simulink model "VCO_15N_2nd_order_2020a_v2"  (R2020b)
settings: Solver=VariableStepAuto  StartTime=0.0  StopTime=5000*clk_p  RelTol=1e-3
values from neighbouring files (symbols this model uses):
  clk_p = 1/clk    (= 5e-09)    [parallel_simulink_test8.m]
  finw = 2*pi*M/(N_in*clk_p)    (= 3374757.73335)    [parallel_simulink_test8.m]
undefined symbols (not defined in the file or in its folder): Amp_in, Bias, gain_DAC
libraries: commsynccomp2 x60, simulink_extras x9, eeGeneralControl x3
(part 1 of 2)
settings Model: SimulationMode=accelerator  Creator=97826  LastModifiedBy=97826
settings SFSimCC: CustomCodeUndefinedFunction=UseInterfaceOnly

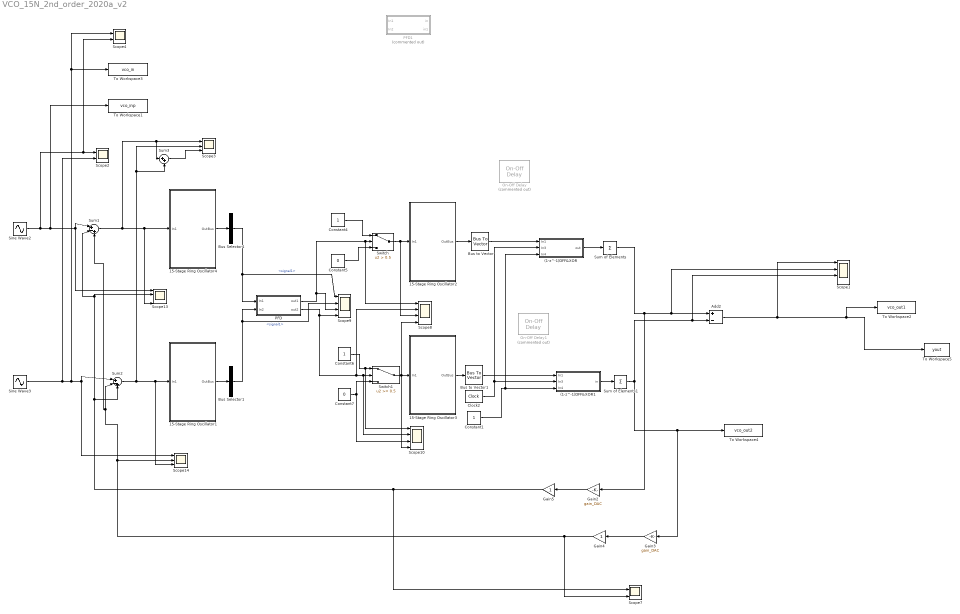
== system VCO_15N_2nd_order_2020a_v2 ==
  (1-z^-1)DFF&XOR : Subsystem  TreatAsAtomicUnit=on
  (1-z^-1)DFF&XOR1 : Subsystem  TreatAsAtomicUnit=on
  15-Stage Ring Oscillator1 : Subsystem
  15-Stage Ring Oscillator2 : Subsystem
  15-Stage Ring Oscillator3 : Subsystem
  15-Stage Ring Oscillator4 : Subsystem
  Add2 : Sum  Inputs=+-
  Bus Selector1 : BusSelector  OutputSignals=signal1
  Bus Selector4 : BusSelector  OutputSignals=signal1
  Bus to Vector : BusToVector
  Bus to Vector1 : BusToVector
  Clock2 : simulink_extras/Flip Flops/Clock  period=clk_p
  Constant1 : Constant
  Constant4 : Constant
  Constant5 : Constant  Value=0
  Constant6 : Constant
  Constant7 : Constant  Value=0
  Gain2 : Gain  Gain=gain_DAC
  Gain3 : Gain  Gain=gain_DAC
  Gain4 : Gain
  Gain5 : Gain
  On-Off Delay : eeGeneralControl/On-Off Delay  Commented=on  LabelModeActiveChoice=Continuous  Td_on=1500e-12  Td_off=1500e-12  IC=0  Ts=0
      settings: SourceProductBaseCode=PS
  On-Off Delay1 : eeGeneralControl/On-Off Delay  Commented=on  LabelModeActiveChoice=Continuous  Td_on=1500e-12  Td_off=1500e-12  IC=0  Ts=0
      settings: SourceProductBaseCode=PS
  PFD : Subsystem  TreatAsAtomicUnit=on
  PFD1 : Subsystem  Commented=on  TreatAsAtomicUnit=on
  Scope{1,8..10,13} (5 alike) : Scope  NumInputPorts=4
  Scope14 : Scope  NumInputPorts=3
  Scope2 : Scope  NumInputPorts=2
  Scope3 : Scope  NumInputPorts=3
  Scope4 : Scope  NumInputPorts=2
  Scope7 : Scope  NumInputPorts=2
  Sine Wave2 : Sin  Amplitude=Amp_in  Bias=Bias  Frequency=finw  SampleTime=0
  Sine Wave3 : Sin  Amplitude=Amp_in  Bias=Bias  Frequency=finw  Phase=pi  SampleTime=0
  Sum of Elements : Sum  Inputs=+  CollapseMode=Specified dimension
  Sum of Elements1 : Sum  Inputs=+  CollapseMode=Specified dimension
  Sum1 : Sum  Inputs=|+-+
  Sum2 : Sum  Inputs=|+-+
  Sum3 : Sum  Inputs=|++
  Switch : Switch  Criteria=u2 > Threshold  Threshold=0.5
  Switch1 : Switch  Threshold=0.5
  To Workspace1 : ToWorkspace  VariableName=vco_inp  SampleTime=-1
  To Workspace2 : ToWorkspace  VariableName=vco_out1  SampleTime=clk_p
  To Workspace3 : ToWorkspace  VariableName=vco_in  SampleTime=-1
  To Workspace4 : ToWorkspace  VariableName=vco_out2  SampleTime=-1
  To Workspace5 : ToWorkspace  VariableName=yout  SampleTime=-1
  wires:
  Sum2/1 -> 15-Stage Ring Oscillator1/1(In1), Scope14/3, Sum3/2, Scope3/2
  Sine Wave3/1 -> Scope4/1, To Workspace3/1, Scope14/1, Sum2/1, Scope2/2
  Gain5/1 -> Sum2/3, Sum1/2, Scope13/2, Scope7/1
  Sine Wave2/1 -> Scope4/2, Scope2/1, To Workspace1/1, Scope13/1, Sum1/1
  Gain4/1 -> Sum1/3, Sum2/2, Scope14/2, Scope7/2
  Gain3/1 -> Gain4/1
  Gain2/1 -> Gain5/1
  Sum1/1 -> Sum3/1, Scope3/1, Scope13/4, 15-Stage Ring Oscillator4/1(In1)
  15-Stage Ring Oscillator4/1(OutBus) -> Bus Selector4/1
  Bus Selector4/1 -> PFD/1(In1), Scope9/1  "<signal1>"
  Bus Selector1/1 -> Scope9/2, PFD/2(In2)  "<signal1>"
  15-Stage Ring Oscillator1/1(OutBus) -> Bus Selector1/1
  Switch/1 -> Scope8/3, 15-Stage Ring Oscillator2/1(In1)
  Constant4/1 -> Switch/1
  Constant5/1 -> Switch/3
  PFD/1(out1) -> Scope9/3, Scope8/1, Switch/2
  Switch1/1 -> 15-Stage Ring Oscillator3/1(In1), Scope8/4, Scope10/4
  Constant7/1 -> Scope10/3, Switch1/3
  Constant6/1 -> Scope10/1, Switch1/1
  PFD/2(out2) -> Scope9/4, Scope8/2, Scope10/2, Switch1/2
  Clock2/1 -> (1-z^-1)DFF&XOR/2(In3), (1-z^-1)DFF&XOR1/2(In3)
  Constant1/1 -> (1-z^-1)DFF&XOR/3(In4), (1-z^-1)DFF&XOR1/3(In4)
  (1-z^-1)DFF&XOR/1(out) -> Sum of Elements/1
  (1-z^-1)DFF&XOR1/1(in) -> Sum of Elements1/1
  Sum of Elements/1 -> Gain2/1, Scope1/2, Add2/1
  Sum of Elements1/1 -> Gain3/1, To Workspace4/1, Scope1/3, Add2/2
  15-Stage Ring Oscillator3/1(OutBus) -> Bus to Vector1/1
  Add2/1 -> Scope1/1, To Workspace2/1, To Workspace5/1
  Sum3/1 -> Scope3/3
  15-Stage Ring Oscillator2/1(OutBus) -> Bus to Vector/1
  Bus to Vector/1 -> (1-z^-1)DFF&XOR/1(In1)
  Bus to Vector1/1 -> (1-z^-1)DFF&XOR1/1(In1)

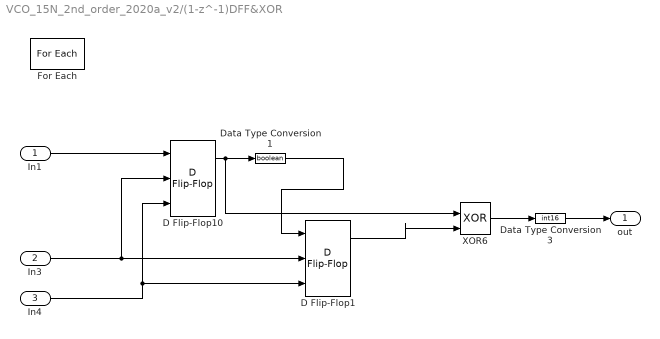
== system VCO_15N_2nd_order_2020a_v2/(1-z^-1)DFF&XOR ==
  In1 : Inport  Partition=on  PartitionDimension=1  PartitionWidth=N_stage  PartitionOffset=0
  In3 : Inport  Port=2
  In4 : Inport  Port=3
  D Flip-Flop1 : simulink_extras/Flip Flops/D Flip-Flop
  D Flip-Flop10 : simulink_extras/Flip Flops/D Flip-Flop
  Data Type Conversion1 : DataTypeConversion  OutDataTypeStr=boolean
  Data Type Conversion3 : DataTypeConversion  OutDataTypeStr=int16
  For Each : ForEach  DisableCoverage=on
  XOR6 : Logic  Operator=XOR  IconShape=distinctive  AllPortsSameDT=off  OutDataTypeStr=boolean
  out : Outport  ConcatenationDimension=1
  wires:
  In3/1 -> D Flip-Flop10/2, D Flip-Flop1/2
  In4/1 -> D Flip-Flop10/3, D Flip-Flop1/3
  Data Type Conversion3/1 -> out/1
  XOR6/1 -> Data Type Conversion3/1
  D Flip-Flop1/1 -> XOR6/2
  In1/1 -> D Flip-Flop10/1
  D Flip-Flop10/1 -> XOR6/1, Data Type Conversion1/1
  Data Type Conversion1/1 -> D Flip-Flop1/1

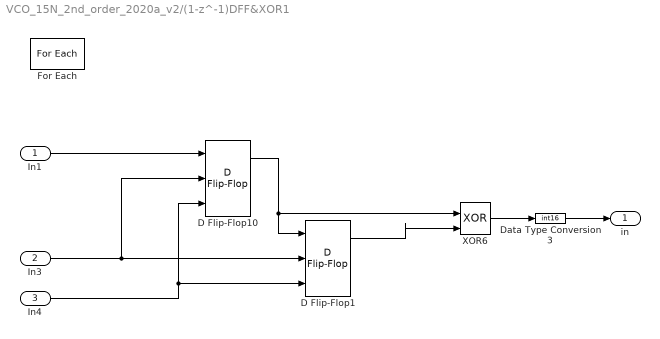
== system VCO_15N_2nd_order_2020a_v2/(1-z^-1)DFF&XOR1 ==
  In1 : Inport  Partition=on  PartitionDimension=1  PartitionWidth=N_stage  PartitionOffset=0
  In3 : Inport  Port=2
  In4 : Inport  Port=3
  D Flip-Flop1 : simulink_extras/Flip Flops/D Flip-Flop
  D Flip-Flop10 : simulink_extras/Flip Flops/D Flip-Flop
  Data Type Conversion3 : DataTypeConversion  OutDataTypeStr=int16
  For Each : ForEach  DisableCoverage=on
  XOR6 : Logic  Operator=XOR  IconShape=distinctive  AllPortsSameDT=off  OutDataTypeStr=boolean
  in : Outport  ConcatenationDimension=1
  wires:
  In3/1 -> D Flip-Flop10/2, D Flip-Flop1/2
  In4/1 -> D Flip-Flop10/3, D Flip-Flop1/3
  Data Type Conversion3/1 -> in/1
  In1/1 -> D Flip-Flop10/1
  XOR6/1 -> Data Type Conversion3/1
  D Flip-Flop1/1 -> XOR6/2
  D Flip-Flop10/1 -> XOR6/1, D Flip-Flop1/1

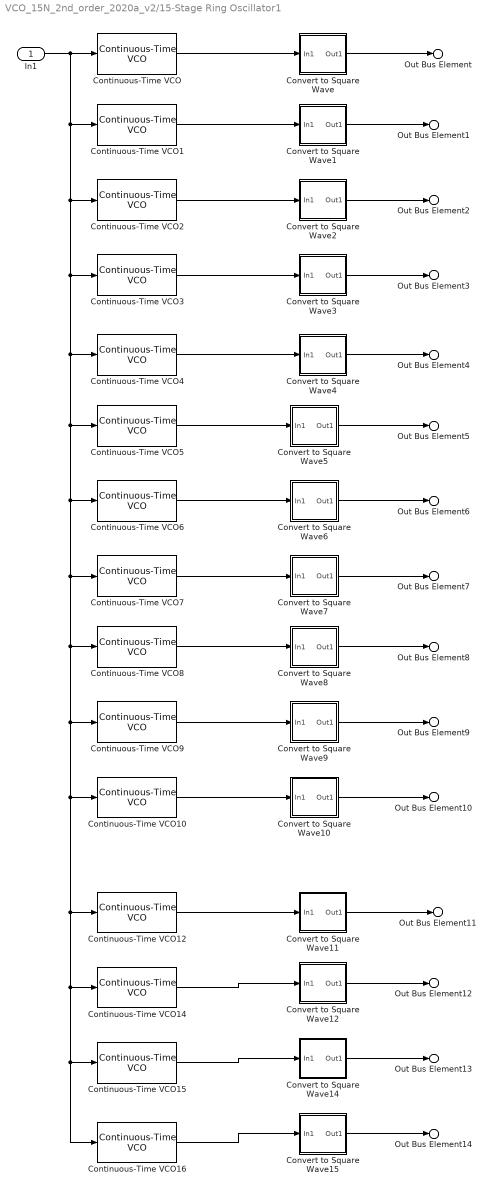
== system VCO_15N_2nd_order_2020a_v2/15-Stage Ring Oscillator1 ==
  In1 : Inport
  Continuous-Time VCO : commsynccomp2/Continuous-Time VCO  Ac=1  Fc=VCO_center_freq1  Kc=KVCO  Ph=1
      settings: SourceProductBaseCode=CM
  Continuous-Time VCO1 : commsynccomp2/Continuous-Time VCO  Ac=1  Fc=VCO_center_freq1  Kc=KVCO  Ph=pi-pi/15+1
      settings: SourceProductBaseCode=CM
  Continuous-Time VCO10 : commsynccomp2/Continuous-Time VCO  Ac=1  Fc=VCO_center_freq1  Kc=KVCO  Ph=-10*pi/15+1
      settings: SourceProductBaseCode=CM
  Continuous-Time VCO12 : commsynccomp2/Continuous-Time VCO  Ac=1  Fc=VCO_center_freq1  Kc=KVCO  Ph=pi-11*pi/15+1
      settings: SourceProductBaseCode=CM
  Continuous-Time VCO14 : commsynccomp2/Continuous-Time VCO  Ac=1  Fc=VCO_center_freq1  Kc=KVCO  Ph=-12*pi/15+1
      settings: SourceProductBaseCode=CM
  Continuous-Time VCO15 : commsynccomp2/Continuous-Time VCO  Ac=1  Fc=VCO_center_freq1  Kc=KVCO  Ph=pi-13*pi/15+1
      settings: SourceProductBaseCode=CM
  Continuous-Time VCO16 : commsynccomp2/Continuous-Time VCO  Ac=1  Fc=VCO_center_freq1  Kc=KVCO  Ph=-14*pi/15+1
      settings: SourceProductBaseCode=CM
  Continuous-Time VCO2 : commsynccomp2/Continuous-Time VCO  Ac=1  Fc=VCO_center_freq1  Kc=KVCO  Ph=-2*pi/15+1
      settings: SourceProductBaseCode=CM
  Continuous-Time VCO3 : commsynccomp2/Continuous-Time VCO  Ac=1  Fc=VCO_center_freq1  Kc=KVCO  Ph=pi-3*pi/15+1
      settings: SourceProductBaseCode=CM
  Continuous-Time VCO4 : commsynccomp2/Continuous-Time VCO  Ac=1  Fc=VCO_center_freq1  Kc=KVCO  Ph=-4*pi/15+1
      settings: SourceProductBaseCode=CM
  Continuous-Time VCO5 : commsynccomp2/Continuous-Time VCO  Ac=1  Fc=VCO_center_freq1  Kc=KVCO  Ph=pi-5*pi/15+1
      settings: SourceProductBaseCode=CM
  Continuous-Time VCO6 : commsynccomp2/Continuous-Time VCO  Ac=1  Fc=VCO_center_freq1  Kc=KVCO  Ph=-6*pi/15+1
      settings: SourceProductBaseCode=CM
  Continuous-Time VCO7 : commsynccomp2/Continuous-Time VCO  Ac=1  Fc=VCO_center_freq1  Kc=KVCO  Ph=pi-7*pi/15+1
      settings: SourceProductBaseCode=CM
  Continuous-Time VCO8 : commsynccomp2/Continuous-Time VCO  Ac=1  Fc=VCO_center_freq1  Kc=KVCO  Ph=-8*pi/15+1
      settings: SourceProductBaseCode=CM
  Continuous-Time VCO9 : commsynccomp2/Continuous-Time VCO  Ac=1  Fc=VCO_center_freq1  Kc=KVCO  Ph=pi-9*pi/15+1
      settings: SourceProductBaseCode=CM
  Convert to Square Wave : Subsystem
  Convert to Square Wave1 : Subsystem
  Convert to Square Wave10 : Subsystem
  Convert to Square Wave11 : Subsystem
  Convert to Square Wave12 : Subsystem
  Convert to Square Wave14 : Subsystem
  Convert to Square Wave15 : Subsystem
  Convert to Square Wave2 : Subsystem
  Convert to Square Wave3 : Subsystem
  Convert to Square Wave4 : Subsystem
  Convert to Square Wave5 : Subsystem
  Convert to Square Wave6 : Subsystem
  Convert to Square Wave7 : Subsystem
  Convert to Square Wave8 : Subsystem
  Convert to Square Wave9 : Subsystem
  Out Bus Element : Outport  PortName=OutBus  Element=signal1
  Out Bus Element1 : Outport  PortName=OutBus  Element=signal2
  Out Bus Element2 : Outport  PortName=OutBus  Element=signal3
  Out Bus Element3 : Outport  PortName=OutBus  Element=signal4
  Out Bus Element4 : Outport  PortName=OutBus  Element=signal5
  Out Bus Element5 : Outport  PortName=OutBus  Element=signal6
  Out Bus Element6 : Outport  PortName=OutBus  Element=signal7
  Out Bus Element7 : Outport  PortName=OutBus  Element=signal8
  Out Bus Element8 : Outport  PortName=OutBus  Element=signal9
  Out Bus Element9 : Outport  PortName=OutBus  Element=signal10
  Out Bus Element10 : Outport  PortName=OutBus  Element=signal11
  Out Bus Element11 : Outport  PortName=OutBus  Element=signal12
  Out Bus Element12 : Outport  PortName=OutBus  Element=signal13
  Out Bus Element13 : Outport  PortName=OutBus  Element=signal14
  Out Bus Element14 : Outport  PortName=OutBus  Element=signal15
  wires:
  Continuous-Time VCO/1 -> Convert to Square Wave/1(In1)
  Continuous-Time VCO1/1 -> Convert to Square Wave1/1(In1)
  Continuous-Time VCO2/1 -> Convert to Square Wave2/1(In1)
  Continuous-Time VCO3/1 -> Convert to Square Wave3/1(In1)
  Continuous-Time VCO4/1 -> Convert to Square Wave4/1(In1)
  Continuous-Time VCO5/1 -> Convert to Square Wave5/1(In1)
  Continuous-Time VCO6/1 -> Convert to Square Wave6/1(In1)
  Continuous-Time VCO7/1 -> Convert to Square Wave7/1(In1)
  Continuous-Time VCO8/1 -> Convert to Square Wave8/1(In1)
  Continuous-Time VCO9/1 -> Convert to Square Wave9/1(In1)
  Continuous-Time VCO10/1 -> Convert to Square Wave10/1(In1)
  Convert to Square Wave/1(Out1) -> Out Bus Element/1
  Convert to Square Wave1/1(Out1) -> Out Bus Element1/1
  Convert to Square Wave2/1(Out1) -> Out Bus Element2/1
  Convert to Square Wave3/1(Out1) -> Out Bus Element3/1
  Convert to Square Wave4/1(Out1) -> Out Bus Element4/1
  Convert to Square Wave5/1(Out1) -> Out Bus Element5/1
  Convert to Square Wave6/1(Out1) -> Out Bus Element6/1
  Convert to Square Wave7/1(Out1) -> Out Bus Element7/1
  Convert to Square Wave8/1(Out1) -> Out Bus Element8/1
  Convert to Square Wave9/1(Out1) -> Out Bus Element9/1
  Convert to Square Wave10/1(Out1) -> Out Bus Element10/1
  Continuous-Time VCO12/1 -> Convert to Square Wave11/1(In1)
  Continuous-Time VCO14/1 -> Convert to Square Wave12/1(In1)
  Continuous-Time VCO15/1 -> Convert to Square Wave14/1(In1)
  Continuous-Time VCO16/1 -> Convert to Square Wave15/1(In1)
  Convert to Square Wave11/1(Out1) -> Out Bus Element11/1
  Convert to Square Wave12/1(Out1) -> Out Bus Element12/1
  Convert to Square Wave14/1(Out1) -> Out Bus Element13/1
  Convert to Square Wave15/1(Out1) -> Out Bus Element14/1
  In1/1 -> Continuous-Time VCO/1, Continuous-Time VCO1/1, Continuous-Time VCO2/1, Continuous-Time VCO3/1, Continuous-Time VCO4/1, Continuous-Time VCO5/1, Continuous-Time VCO6/1, Continuous-Time VCO7/1, Continuous-Time VCO8/1, Continuous-Time VCO9/1, Continuous-Time VCO12/1, Continuous-Time VCO14/1, Continuous-Time VCO15/1, Continuous-Time VCO16/1, Continuous-Time VCO10/1

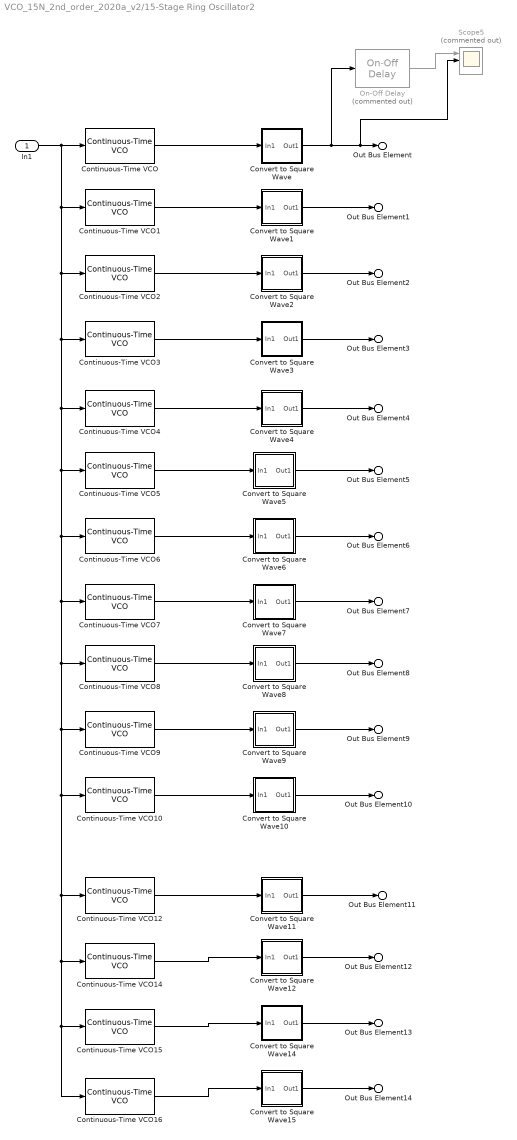
== system VCO_15N_2nd_order_2020a_v2/15-Stage Ring Oscillator2 ==
  In1 : Inport
  Continuous-Time VCO : commsynccomp2/Continuous-Time VCO  Ac=1  Fc=VCO_center_freq  Kc=KVCO2  Ph=1
      settings: SourceProductBaseCode=CM
  Continuous-Time VCO1 : commsynccomp2/Continuous-Time VCO  Ac=1  Fc=VCO_center_freq  Kc=KVCO2  Ph=pi-pi/15+1
      settings: SourceProductBaseCode=CM
  Continuous-Time VCO10 : commsynccomp2/Continuous-Time VCO  Ac=1  Fc=VCO_center_freq  Kc=KVCO2  Ph=-10*pi/15+1
      settings: SourceProductBaseCode=CM
  Continuous-Time VCO12 : commsynccomp2/Continuous-Time VCO  Ac=1  Fc=VCO_center_freq  Kc=KVCO2  Ph=pi-11*pi/15+1
      settings: SourceProductBaseCode=CM
  Continuous-Time VCO14 : commsynccomp2/Continuous-Time VCO  Ac=1  Fc=VCO_center_freq  Kc=KVCO2  Ph=-12*pi/15+1
      settings: SourceProductBaseCode=CM
  Continuous-Time VCO15 : commsynccomp2/Continuous-Time VCO  Ac=1  Fc=VCO_center_freq  Kc=KVCO2  Ph=pi-13*pi/15+1
      settings: SourceProductBaseCode=CM
  Continuous-Time VCO16 : commsynccomp2/Continuous-Time VCO  Ac=1  Fc=VCO_center_freq  Kc=KVCO2  Ph=-14*pi/15+1
      settings: SourceProductBaseCode=CM
  Continuous-Time VCO2 : commsynccomp2/Continuous-Time VCO  Ac=1  Fc=VCO_center_freq  Kc=KVCO2  Ph=-2*pi/15+1
      settings: SourceProductBaseCode=CM
  Continuous-Time VCO3 : commsynccomp2/Continuous-Time VCO  Ac=1  Fc=VCO_center_freq  Kc=KVCO2  Ph=pi-3*pi/15+1
      settings: SourceProductBaseCode=CM
  Continuous-Time VCO4 : commsynccomp2/Continuous-Time VCO  Ac=1  Fc=VCO_center_freq  Kc=KVCO2  Ph=-4*pi/15+1
      settings: SourceProductBaseCode=CM
  Continuous-Time VCO5 : commsynccomp2/Continuous-Time VCO  Ac=1  Fc=VCO_center_freq  Kc=KVCO2  Ph=pi-5*pi/15+1
      settings: SourceProductBaseCode=CM
  Continuous-Time VCO6 : commsynccomp2/Continuous-Time VCO  Ac=1  Fc=VCO_center_freq  Kc=KVCO2  Ph=-6*pi/15+1
      settings: SourceProductBaseCode=CM
  Continuous-Time VCO7 : commsynccomp2/Continuous-Time VCO  Ac=1  Fc=VCO_center_freq  Kc=KVCO2  Ph=pi-7*pi/15+1
      settings: SourceProductBaseCode=CM
  Continuous-Time VCO8 : commsynccomp2/Continuous-Time VCO  Ac=1  Fc=VCO_center_freq  Kc=KVCO2  Ph=-8*pi/15+1
      settings: SourceProductBaseCode=CM
  Continuous-Time VCO9 : commsynccomp2/Continuous-Time VCO  Ac=1  Fc=VCO_center_freq  Kc=KVCO2  Ph=pi-9*pi/15+1
      settings: SourceProductBaseCode=CM
  Convert to Square Wave : Subsystem
  Convert to Square Wave1 : Subsystem
  Convert to Square Wave10 : Subsystem
  Convert to Square Wave11 : Subsystem
  Convert to Square Wave12 : Subsystem
  Convert to Square Wave14 : Subsystem
  Convert to Square Wave15 : Subsystem
  Convert to Square Wave2 : Subsystem
  Convert to Square Wave3 : Subsystem
  Convert to Square Wave4 : Subsystem
  Convert to Square Wave5 : Subsystem
  Convert to Square Wave6 : Subsystem
  Convert to Square Wave7 : Subsystem
  Convert to Square Wave8 : Subsystem
  Convert to Square Wave9 : Subsystem
  On-Off Delay : eeGeneralControl/On-Off Delay  Commented=on  LabelModeActiveChoice=Continuous  Td_on=100e-12  Td_off=100e-12  IC=0  Ts=0
      settings: SourceProductBaseCode=PS
  Scope5 : Scope  Commented=on  NumInputPorts=3
  Out Bus Element : Outport  PortName=OutBus  Element=signal1
  Out Bus Element1 : Outport  PortName=OutBus  Element=signal2
  Out Bus Element2 : Outport  PortName=OutBus  Element=signal3
  Out Bus Element3 : Outport  PortName=OutBus  Element=signal4
  Out Bus Element4 : Outport  PortName=OutBus  Element=signal5
  Out Bus Element5 : Outport  PortName=OutBus  Element=signal6
  Out Bus Element6 : Outport  PortName=OutBus  Element=signal7
  Out Bus Element7 : Outport  PortName=OutBus  Element=signal8
  Out Bus Element8 : Outport  PortName=OutBus  Element=signal9
  Out Bus Element9 : Outport  PortName=OutBus  Element=signal10
  Out Bus Element10 : Outport  PortName=OutBus  Element=signal11
  Out Bus Element11 : Outport  PortName=OutBus  Element=signal12
  Out Bus Element12 : Outport  PortName=OutBus  Element=signal13
  Out Bus Element13 : Outport  PortName=OutBus  Element=signal14
  Out Bus Element14 : Outport  PortName=OutBus  Element=signal15
  wires:
  Continuous-Time VCO/1 -> Convert to Square Wave/1(In1)
  Continuous-Time VCO1/1 -> Convert to Square Wave1/1(In1)
  Continuous-Time VCO2/1 -> Convert to Square Wave2/1(In1)
  Continuous-Time VCO3/1 -> Convert to Square Wave3/1(In1)
  Continuous-Time VCO4/1 -> Convert to Square Wave4/1(In1)
  Continuous-Time VCO5/1 -> Convert to Square Wave5/1(In1)
  Continuous-Time VCO6/1 -> Convert to Square Wave6/1(In1)
  Continuous-Time VCO7/1 -> Convert to Square Wave7/1(In1)
  Continuous-Time VCO8/1 -> Convert to Square Wave8/1(In1)
  Continuous-Time VCO9/1 -> Convert to Square Wave9/1(In1)
  Continuous-Time VCO10/1 -> Convert to Square Wave10/1(In1)
  Convert to Square Wave1/1(Out1) -> Out Bus Element1/1
  Convert to Square Wave2/1(Out1) -> Out Bus Element2/1
  Convert to Square Wave3/1(Out1) -> Out Bus Element3/1
  Convert to Square Wave4/1(Out1) -> Out Bus Element4/1
  Convert to Square Wave5/1(Out1) -> Out Bus Element5/1
  Convert to Square Wave6/1(Out1) -> Out Bus Element6/1
  Convert to Square Wave7/1(Out1) -> Out Bus Element7/1
  Convert to Square Wave8/1(Out1) -> Out Bus Element8/1
  Convert to Square Wave9/1(Out1) -> Out Bus Element9/1
  Convert to Square Wave10/1(Out1) -> Out Bus Element10/1
  Continuous-Time VCO12/1 -> Convert to Square Wave11/1(In1)
  Continuous-Time VCO14/1 -> Convert to Square Wave12/1(In1)
  Continuous-Time VCO15/1 -> Convert to Square Wave14/1(In1)
  Continuous-Time VCO16/1 -> Convert to Square Wave15/1(In1)
  Convert to Square Wave11/1(Out1) -> Out Bus Element11/1
  Convert to Square Wave12/1(Out1) -> Out Bus Element12/1
  Convert to Square Wave14/1(Out1) -> Out Bus Element13/1
  Convert to Square Wave15/1(Out1) -> Out Bus Element14/1
  In1/1 -> Continuous-Time VCO/1, Continuous-Time VCO1/1, Continuous-Time VCO2/1, Continuous-Time VCO3/1, Continuous-Time VCO4/1, Continuous-Time VCO5/1, Continuous-Time VCO6/1, Continuous-Time VCO7/1, Continuous-Time VCO8/1, Continuous-Time VCO9/1, Continuous-Time VCO12/1, Continuous-Time VCO14/1, Continuous-Time VCO15/1, Continuous-Time VCO16/1, Continuous-Time VCO10/1
  On-Off Delay/1 -> Scope5/1
  Convert to Square Wave/1(Out1) -> On-Off Delay/1, Scope5/2, Out Bus Element/1

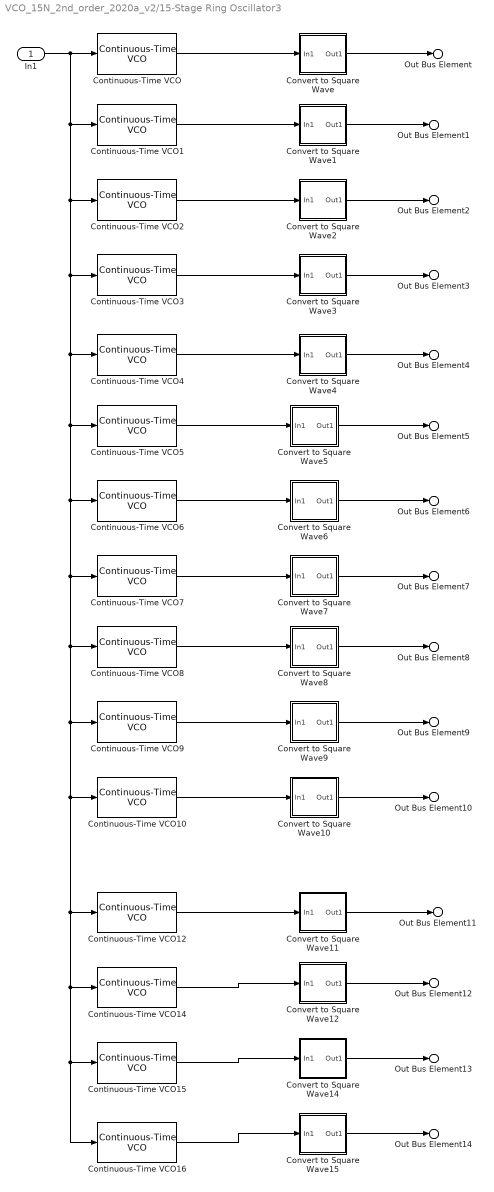
== system VCO_15N_2nd_order_2020a_v2/15-Stage Ring Oscillator3 ==
  In1 : Inport
  Continuous-Time VCO : commsynccomp2/Continuous-Time VCO  Ac=1  Fc=VCO_center_freq  Kc=KVCO2  Ph=1
      settings: SourceProductBaseCode=CM
  Continuous-Time VCO1 : commsynccomp2/Continuous-Time VCO  Ac=1  Fc=VCO_center_freq  Kc=KVCO2  Ph=pi-pi/15+1
      settings: SourceProductBaseCode=CM
  Continuous-Time VCO10 : commsynccomp2/Continuous-Time VCO  Ac=1  Fc=VCO_center_freq  Kc=KVCO2  Ph=-10*pi/15+1
      settings: SourceProductBaseCode=CM
  Continuous-Time VCO12 : commsynccomp2/Continuous-Time VCO  Ac=1  Fc=VCO_center_freq  Kc=KVCO2  Ph=pi-11*pi/15+1
      settings: SourceProductBaseCode=CM
  Continuous-Time VCO14 : commsynccomp2/Continuous-Time VCO  Ac=1  Fc=VCO_center_freq  Kc=KVCO2  Ph=-12*pi/15+1
      settings: SourceProductBaseCode=CM
  Continuous-Time VCO15 : commsynccomp2/Continuous-Time VCO  Ac=1  Fc=VCO_center_freq  Kc=KVCO2  Ph=pi-13*pi/15+1
      settings: SourceProductBaseCode=CM
  Continuous-Time VCO16 : commsynccomp2/Continuous-Time VCO  Ac=1  Fc=VCO_center_freq  Kc=KVCO2  Ph=-14*pi/15+1
      settings: SourceProductBaseCode=CM
  Continuous-Time VCO2 : commsynccomp2/Continuous-Time VCO  Ac=1  Fc=VCO_center_freq  Kc=KVCO2  Ph=-2*pi/15+1
      settings: SourceProductBaseCode=CM
  Continuous-Time VCO3 : commsynccomp2/Continuous-Time VCO  Ac=1  Fc=VCO_center_freq  Kc=KVCO2  Ph=pi-3*pi/15+1
      settings: SourceProductBaseCode=CM
  Continuous-Time VCO4 : commsynccomp2/Continuous-Time VCO  Ac=1  Fc=VCO_center_freq  Kc=KVCO2  Ph=-4*pi/15+1
      settings: SourceProductBaseCode=CM
  Continuous-Time VCO5 : commsynccomp2/Continuous-Time VCO  Ac=1  Fc=VCO_center_freq  Kc=KVCO2  Ph=pi-5*pi/15+1
      settings: SourceProductBaseCode=CM
  Continuous-Time VCO6 : commsynccomp2/Continuous-Time VCO  Ac=1  Fc=VCO_center_freq  Kc=KVCO2  Ph=-6*pi/15+1
      settings: SourceProductBaseCode=CM
  Continuous-Time VCO7 : commsynccomp2/Continuous-Time VCO  Ac=1  Fc=VCO_center_freq  Kc=KVCO2  Ph=pi-7*pi/15+1
      settings: SourceProductBaseCode=CM
  Continuous-Time VCO8 : commsynccomp2/Continuous-Time VCO  Ac=1  Fc=VCO_center_freq  Kc=KVCO2  Ph=-8*pi/15+1
      settings: SourceProductBaseCode=CM
  Continuous-Time VCO9 : commsynccomp2/Continuous-Time VCO  Ac=1  Fc=VCO_center_freq  Kc=KVCO2  Ph=pi-9*pi/15+1
      settings: SourceProductBaseCode=CM
  Convert to Square Wave : Subsystem
  Convert to Square Wave1 : Subsystem
  Convert to Square Wave10 : Subsystem
  Convert to Square Wave11 : Subsystem
  Convert to Square Wave12 : Subsystem
  Convert to Square Wave14 : Subsystem
  Convert to Square Wave15 : Subsystem
  Convert to Square Wave2 : Subsystem
  Convert to Square Wave3 : Subsystem
  Convert to Square Wave4 : Subsystem
  Convert to Square Wave5 : Subsystem
  Convert to Square Wave6 : Subsystem
  Convert to Square Wave7 : Subsystem
  Convert to Square Wave8 : Subsystem
  Convert to Square Wave9 : Subsystem
  Out Bus Element : Outport  PortName=OutBus  Element=signal1
  Out Bus Element1 : Outport  PortName=OutBus  Element=signal2
  Out Bus Element2 : Outport  PortName=OutBus  Element=signal3
  Out Bus Element3 : Outport  PortName=OutBus  Element=signal4
  Out Bus Element4 : Outport  PortName=OutBus  Element=signal5
  Out Bus Element5 : Outport  PortName=OutBus  Element=signal6
  Out Bus Element6 : Outport  PortName=OutBus  Element=signal7
  Out Bus Element7 : Outport  PortName=OutBus  Element=signal8
  Out Bus Element8 : Outport  PortName=OutBus  Element=signal9
  Out Bus Element9 : Outport  PortName=OutBus  Element=signal10
  Out Bus Element10 : Outport  PortName=OutBus  Element=signal11
  Out Bus Element11 : Outport  PortName=OutBus  Element=signal12
  Out Bus Element12 : Outport  PortName=OutBus  Element=signal13
  Out Bus Element13 : Outport  PortName=OutBus  Element=signal14
  Out Bus Element14 : Outport  PortName=OutBus  Element=signal15
  wires:
  Continuous-Time VCO/1 -> Convert to Square Wave/1(In1)
  Continuous-Time VCO1/1 -> Convert to Square Wave1/1(In1)
  Continuous-Time VCO2/1 -> Convert to Square Wave2/1(In1)
  Continuous-Time VCO3/1 -> Convert to Square Wave3/1(In1)
  Continuous-Time VCO4/1 -> Convert to Square Wave4/1(In1)
  Continuous-Time VCO5/1 -> Convert to Square Wave5/1(In1)
  Continuous-Time VCO6/1 -> Convert to Square Wave6/1(In1)
  Continuous-Time VCO7/1 -> Convert to Square Wave7/1(In1)
  Continuous-Time VCO8/1 -> Convert to Square Wave8/1(In1)
  Continuous-Time VCO9/1 -> Convert to Square Wave9/1(In1)
  Continuous-Time VCO10/1 -> Convert to Square Wave10/1(In1)
  Convert to Square Wave/1(Out1) -> Out Bus Element/1
  Convert to Square Wave1/1(Out1) -> Out Bus Element1/1
  Convert to Square Wave2/1(Out1) -> Out Bus Element2/1
  Convert to Square Wave3/1(Out1) -> Out Bus Element3/1
  Convert to Square Wave4/1(Out1) -> Out Bus Element4/1
  Convert to Square Wave5/1(Out1) -> Out Bus Element5/1
  Convert to Square Wave6/1(Out1) -> Out Bus Element6/1
  Convert to Square Wave7/1(Out1) -> Out Bus Element7/1
  Convert to Square Wave8/1(Out1) -> Out Bus Element8/1
  Convert to Square Wave9/1(Out1) -> Out Bus Element9/1
  Convert to Square Wave10/1(Out1) -> Out Bus Element10/1
  Continuous-Time VCO12/1 -> Convert to Square Wave11/1(In1)
  Continuous-Time VCO14/1 -> Convert to Square Wave12/1(In1)
  Continuous-Time VCO15/1 -> Convert to Square Wave14/1(In1)
  Continuous-Time VCO16/1 -> Convert to Square Wave15/1(In1)
  Convert to Square Wave11/1(Out1) -> Out Bus Element11/1
  Convert to Square Wave12/1(Out1) -> Out Bus Element12/1
  Convert to Square Wave14/1(Out1) -> Out Bus Element13/1
  Convert to Square Wave15/1(Out1) -> Out Bus Element14/1
  In1/1 -> Continuous-Time VCO/1, Continuous-Time VCO1/1, Continuous-Time VCO2/1, Continuous-Time VCO3/1, Continuous-Time VCO4/1, Continuous-Time VCO5/1, Continuous-Time VCO6/1, Continuous-Time VCO7/1, Continuous-Time VCO8/1, Continuous-Time VCO9/1, Continuous-Time VCO12/1, Continuous-Time VCO14/1, Continuous-Time VCO15/1, Continuous-Time VCO16/1, Continuous-Time VCO10/1

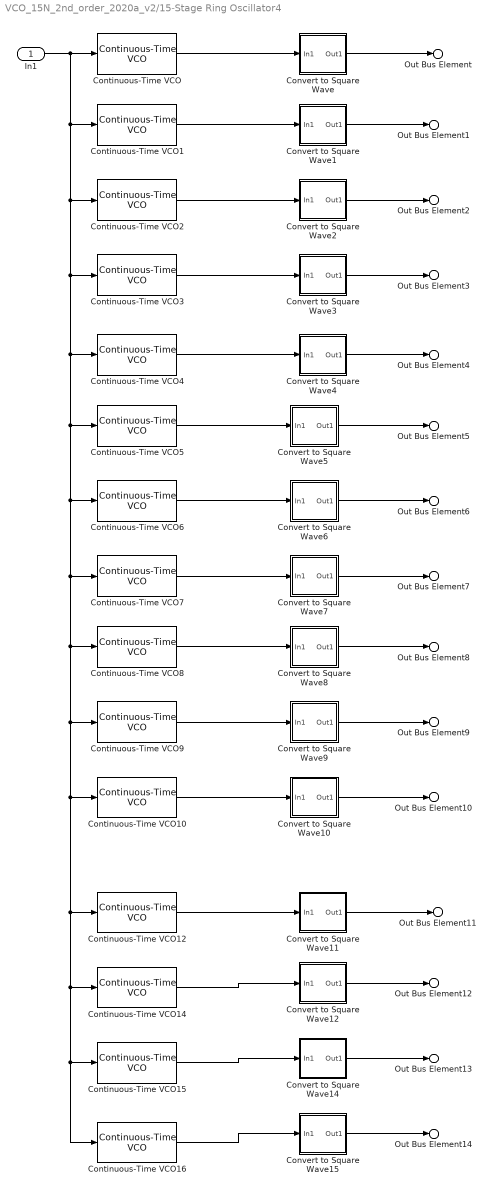
== system VCO_15N_2nd_order_2020a_v2/15-Stage Ring Oscillator4 ==
  In1 : Inport
  Continuous-Time VCO : commsynccomp2/Continuous-Time VCO  Ac=1  Fc=VCO_center_freq1  Kc=KVCO  Ph=1
      settings: SourceProductBaseCode=CM
  Continuous-Time VCO1 : commsynccomp2/Continuous-Time VCO  Ac=1  Fc=VCO_center_freq1  Kc=KVCO  Ph=pi-pi/15+1
      settings: SourceProductBaseCode=CM
  Continuous-Time VCO10 : commsynccomp2/Continuous-Time VCO  Ac=1  Fc=VCO_center_freq1  Kc=KVCO  Ph=-10*pi/15+1
      settings: SourceProductBaseCode=CM
  Continuous-Time VCO12 : commsynccomp2/Continuous-Time VCO  Ac=1  Fc=VCO_center_freq1  Kc=KVCO  Ph=pi-11*pi/15+1
      settings: SourceProductBaseCode=CM
  Continuous-Time VCO14 : commsynccomp2/Continuous-Time VCO  Ac=1  Fc=VCO_center_freq1  Kc=KVCO  Ph=-12*pi/15+1
      settings: SourceProductBaseCode=CM
  Continuous-Time VCO15 : commsynccomp2/Continuous-Time VCO  Ac=1  Fc=VCO_center_freq1  Kc=KVCO  Ph=pi-13*pi/15+1
      settings: SourceProductBaseCode=CM
  Continuous-Time VCO16 : commsynccomp2/Continuous-Time VCO  Ac=1  Fc=VCO_center_freq1  Kc=KVCO  Ph=-14*pi/15+1
      settings: SourceProductBaseCode=CM
  Continuous-Time VCO2 : commsynccomp2/Continuous-Time VCO  Ac=1  Fc=VCO_center_freq1  Kc=KVCO  Ph=-2*pi/15+1
      settings: SourceProductBaseCode=CM
  Continuous-Time VCO3 : commsynccomp2/Continuous-Time VCO  Ac=1  Fc=VCO_center_freq1  Kc=KVCO  Ph=pi-3*pi/15+1
      settings: SourceProductBaseCode=CM
  Continuous-Time VCO4 : commsynccomp2/Continuous-Time VCO  Ac=1  Fc=VCO_center_freq1  Kc=KVCO  Ph=-4*pi/15+1
      settings: SourceProductBaseCode=CM
  Continuous-Time VCO5 : commsynccomp2/Continuous-Time VCO  Ac=1  Fc=VCO_center_freq1  Kc=KVCO  Ph=pi-5*pi/15+1
      settings: SourceProductBaseCode=CM
  Continuous-Time VCO6 : commsynccomp2/Continuous-Time VCO  Ac=1  Fc=VCO_center_freq1  Kc=KVCO  Ph=-6*pi/15+1
      settings: SourceProductBaseCode=CM
  Continuous-Time VCO7 : commsynccomp2/Continuous-Time VCO  Ac=1  Fc=VCO_center_freq1  Kc=KVCO  Ph=pi-7*pi/15+1
      settings: SourceProductBaseCode=CM
  Continuous-Time VCO8 : commsynccomp2/Continuous-Time VCO  Ac=1  Fc=VCO_center_freq1  Kc=KVCO  Ph=-8*pi/15+1
      settings: SourceProductBaseCode=CM
  Continuous-Time VCO9 : commsynccomp2/Continuous-Time VCO  Ac=1  Fc=VCO_center_freq1  Kc=KVCO  Ph=pi-9*pi/15+1
      settings: SourceProductBaseCode=CM
  Convert to Square Wave : Subsystem
  Convert to Square Wave1 : Subsystem
  Convert to Square Wave10 : Subsystem
  Convert to Square Wave11 : Subsystem
  Convert to Square Wave12 : Subsystem
  Convert to Square Wave14 : Subsystem
  Convert to Square Wave15 : Subsystem
  Convert to Square Wave2 : Subsystem
  Convert to Square Wave3 : Subsystem
  Convert to Square Wave4 : Subsystem
  Convert to Square Wave5 : Subsystem
  Convert to Square Wave6 : Subsystem
  Convert to Square Wave7 : Subsystem
  Convert to Square Wave8 : Subsystem
  Convert to Square Wave9 : Subsystem
  Out Bus Element : Outport  PortName=OutBus  Element=signal1
  Out Bus Element1 : Outport  PortName=OutBus  Element=signal2
  Out Bus Element2 : Outport  PortName=OutBus  Element=signal3
  Out Bus Element3 : Outport  PortName=OutBus  Element=signal4
  Out Bus Element4 : Outport  PortName=OutBus  Element=signal5
  Out Bus Element5 : Outport  PortName=OutBus  Element=signal6
  Out Bus Element6 : Outport  PortName=OutBus  Element=signal7
  Out Bus Element7 : Outport  PortName=OutBus  Element=signal8
  Out Bus Element8 : Outport  PortName=OutBus  Element=signal9
  Out Bus Element9 : Outport  PortName=OutBus  Element=signal10
  Out Bus Element10 : Outport  PortName=OutBus  Element=signal11
  Out Bus Element11 : Outport  PortName=OutBus  Element=signal12
  Out Bus Element12 : Outport  PortName=OutBus  Element=signal13
  Out Bus Element13 : Outport  PortName=OutBus  Element=signal14
  Out Bus Element14 : Outport  PortName=OutBus  Element=signal15
  wires:
  Continuous-Time VCO/1 -> Convert to Square Wave/1(In1)
  Continuous-Time VCO1/1 -> Convert to Square Wave1/1(In1)
  Continuous-Time VCO2/1 -> Convert to Square Wave2/1(In1)
  Continuous-Time VCO3/1 -> Convert to Square Wave3/1(In1)
  Continuous-Time VCO4/1 -> Convert to Square Wave4/1(In1)
  Continuous-Time VCO5/1 -> Convert to Square Wave5/1(In1)
  Continuous-Time VCO6/1 -> Convert to Square Wave6/1(In1)
  Continuous-Time VCO7/1 -> Convert to Square Wave7/1(In1)
  Continuous-Time VCO8/1 -> Convert to Square Wave8/1(In1)
  Continuous-Time VCO9/1 -> Convert to Square Wave9/1(In1)
  Continuous-Time VCO10/1 -> Convert to Square Wave10/1(In1)
  Convert to Square Wave/1(Out1) -> Out Bus Element/1
  Convert to Square Wave1/1(Out1) -> Out Bus Element1/1
  Convert to Square Wave2/1(Out1) -> Out Bus Element2/1
  Convert to Square Wave3/1(Out1) -> Out Bus Element3/1
  Convert to Square Wave4/1(Out1) -> Out Bus Element4/1
  Convert to Square Wave5/1(Out1) -> Out Bus Element5/1
  Convert to Square Wave6/1(Out1) -> Out Bus Element6/1
  Convert to Square Wave7/1(Out1) -> Out Bus Element7/1
  Convert to Square Wave8/1(Out1) -> Out Bus Element8/1
  Convert to Square Wave9/1(Out1) -> Out Bus Element9/1
  Convert to Square Wave10/1(Out1) -> Out Bus Element10/1
  Continuous-Time VCO12/1 -> Convert to Square Wave11/1(In1)
  Continuous-Time VCO14/1 -> Convert to Square Wave12/1(In1)
  Continuous-Time VCO15/1 -> Convert to Square Wave14/1(In1)
  Continuous-Time VCO16/1 -> Convert to Square Wave15/1(In1)
  Convert to Square Wave11/1(Out1) -> Out Bus Element11/1
  Convert to Square Wave12/1(Out1) -> Out Bus Element12/1
  Convert to Square Wave14/1(Out1) -> Out Bus Element13/1
  Convert to Square Wave15/1(Out1) -> Out Bus Element14/1
  In1/1 -> Continuous-Time VCO/1, Continuous-Time VCO1/1, Continuous-Time VCO2/1, Continuous-Time VCO3/1, Continuous-Time VCO4/1, Continuous-Time VCO5/1, Continuous-Time VCO6/1, Continuous-Time VCO7/1, Continuous-Time VCO8/1, Continuous-Time VCO9/1, Continuous-Time VCO12/1, Continuous-Time VCO14/1, Continuous-Time VCO15/1, Continuous-Time VCO16/1, Continuous-Time VCO10/1

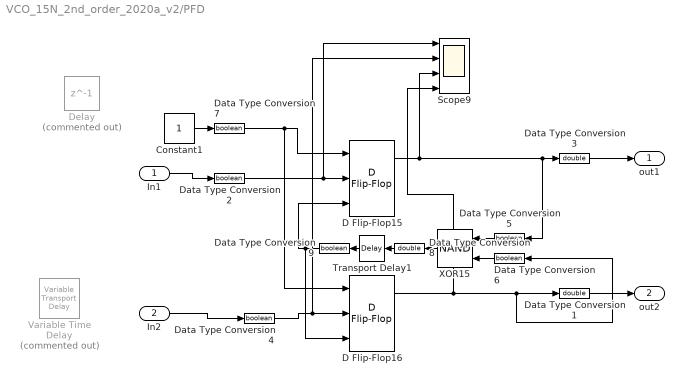
== system VCO_15N_2nd_order_2020a_v2/PFD ==
  In1 : Inport
  In2 : Inport  Port=2
  Constant1 : Constant
  D Flip-Flop15 : simulink_extras/Flip Flops/D Flip-Flop
  D Flip-Flop16 : simulink_extras/Flip Flops/D Flip-Flop
  Data Type Conversion1 : DataTypeConversion  OutDataTypeStr=double
  Data Type Conversion{2,4..7,9} (6 alike) : DataTypeConversion  OutDataTypeStr=boolean
  Data Type Conversion3 : DataTypeConversion  OutDataTypeStr=double
  Data Type Conversion8 : DataTypeConversion  OutDataTypeStr=double
  Delay : Delay  Commented=on  DelayLength=1  InitialCondition=0
  Scope9 : Scope  NumInputPorts=4
  Transport Delay1 : TransportDelay  DelayTime=0.2e-9
  Variable Time Delay : VariableTransportDelay  Commented=on  MaximumDelay=10
  XOR15 : Logic  Operator=NAND  IconShape=distinctive  AllPortsSameDT=off  OutDataTypeStr=boolean
  out1 : Outport
  out2 : Outport  Port=2
  wires:
  Data Type Conversion3/1 -> out1/1
  D Flip-Flop16/1 -> Scope9/4, Data Type Conversion6/1, Data Type Conversion1/1
  D Flip-Flop15/1 -> Scope9/3, Data Type Conversion5/1, Data Type Conversion3/1
  Data Type Conversion1/1 -> out2/1
  Data Type Conversion2/1 -> Scope9/1, D Flip-Flop15/2
  In1/1 -> Data Type Conversion2/1
  Data Type Conversion4/1 -> Scope9/2, D Flip-Flop16/2
  In2/1 -> Data Type Conversion4/1
  Data Type Conversion5/1 -> XOR15/1
  Data Type Conversion6/1 -> XOR15/2
  Constant1/1 -> Data Type Conversion7/1
  Data Type Conversion7/1 -> D Flip-Flop16/1, D Flip-Flop15/1
  Data Type Conversion8/1 -> Transport Delay1/1
  XOR15/1 -> Data Type Conversion8/1
  Transport Delay1/1 -> Data Type Conversion9/1
  Data Type Conversion9/1 -> D Flip-Flop15/3, D Flip-Flop16/3

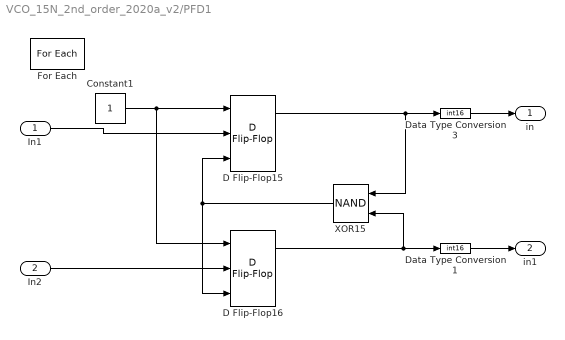
== system VCO_15N_2nd_order_2020a_v2/PFD1 ==
  In1 : Inport  Partition=on  PartitionDimension=1  PartitionWidth=N_stage  PartitionOffset=0
  In2 : Inport  Port=2  Partition=on  PartitionDimension=1  PartitionWidth=N_stage  PartitionOffset=0
  Constant1 : Constant
  D Flip-Flop15 : simulink_extras/Flip Flops/D Flip-Flop
  D Flip-Flop16 : simulink_extras/Flip Flops/D Flip-Flop
  Data Type Conversion1 : DataTypeConversion  OutDataTypeStr=int16
  Data Type Conversion3 : DataTypeConversion  OutDataTypeStr=int16
  For Each : ForEach  DisableCoverage=on
  XOR15 : Logic  Operator=NAND  IconShape=distinctive  AllPortsSameDT=off  OutDataTypeStr=boolean
  in : Outport  ConcatenationDimension=1
  in1 : Outport  Port=2  ConcatenationDimension=1
  wires:
  Data Type Conversion3/1 -> in/1
  D Flip-Flop16/1 -> Data Type Conversion1/1, XOR15/2
  Constant1/1 -> D Flip-Flop15/1, D Flip-Flop16/1
  XOR15/1 -> D Flip-Flop16/3, D Flip-Flop15/3
  D Flip-Flop15/1 -> Data Type Conversion3/1, XOR15/1
  In1/1 -> D Flip-Flop15/2
  In2/1 -> D Flip-Flop16/2
  Data Type Conversion1/1 -> in1/1

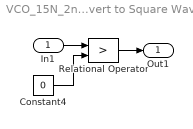
== system VCO_15N_2nd_order_2020a_v2/15-Stage Ring Oscillator1/Convert to Square Wave ==
  In1 : Inport
  Constant4 : Constant  Value=0
  Relational Operator : RelationalOperator  Operator=>  RndMeth=Nearest  InputSameDT=on
  Out1 : Outport
  wires:
  Relational Operator/1 -> Out1/1
  In1/1 -> Relational Operator/1
  Constant4/1 -> Relational Operator/2

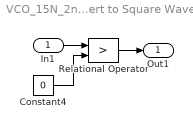
== system VCO_15N_2nd_order_2020a_v2/15-Stage Ring Oscillator1/Convert to Square Wave1 ==
  In1 : Inport
  Constant4 : Constant  Value=0
  Relational Operator : RelationalOperator  Operator=>  RndMeth=Nearest  InputSameDT=on
  Out1 : Outport
  wires:
  Relational Operator/1 -> Out1/1
  In1/1 -> Relational Operator/1
  Constant4/1 -> Relational Operator/2

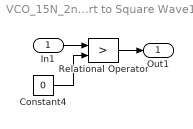
== system VCO_15N_2nd_order_2020a_v2/15-Stage Ring Oscillator1/Convert to Square Wave10 ==
  In1 : Inport
  Constant4 : Constant  Value=0
  Relational Operator : RelationalOperator  Operator=>  RndMeth=Nearest  InputSameDT=on
  Out1 : Outport
  wires:
  Relational Operator/1 -> Out1/1
  In1/1 -> Relational Operator/1
  Constant4/1 -> Relational Operator/2

== system VCO_15N_2nd_order_2020a_v2/15-Stage Ring Oscillator1/Convert to Square Wave11 ==
  In1 : Inport
  Constant4 : Constant  Value=0
  Relational Operator : RelationalOperator  Operator=>  RndMeth=Nearest  InputSameDT=on
  Out1 : Outport
  wires:
  Relational Operator/1 -> Out1/1
  In1/1 -> Relational Operator/1
  Constant4/1 -> Relational Operator/2

== system VCO_15N_2nd_order_2020a_v2/15-Stage Ring Oscillator1/Convert to Square Wave12 ==
  In1 : Inport
  Constant4 : Constant  Value=0
  Relational Operator : RelationalOperator  Operator=>  RndMeth=Nearest  InputSameDT=on
  Out1 : Outport
  wires:
  Relational Operator/1 -> Out1/1
  In1/1 -> Relational Operator/1
  Constant4/1 -> Relational Operator/2

== system VCO_15N_2nd_order_2020a_v2/15-Stage Ring Oscillator1/Convert to Square Wave14 ==
  In1 : Inport
  Constant4 : Constant  Value=0
  Relational Operator : RelationalOperator  Operator=>  RndMeth=Nearest  InputSameDT=on
  Out1 : Outport
  wires:
  Relational Operator/1 -> Out1/1
  In1/1 -> Relational Operator/1
  Constant4/1 -> Relational Operator/2

== system VCO_15N_2nd_order_2020a_v2/15-Stage Ring Oscillator1/Convert to Square Wave15 ==
  In1 : Inport
  Constant4 : Constant  Value=0
  Relational Operator : RelationalOperator  Operator=>  RndMeth=Nearest  InputSameDT=on
  Out1 : Outport
  wires:
  Relational Operator/1 -> Out1/1
  In1/1 -> Relational Operator/1
  Constant4/1 -> Relational Operator/2

== system VCO_15N_2nd_order_2020a_v2/15-Stage Ring Oscillator1/Convert to Square Wave2 ==
  In1 : Inport
  Constant4 : Constant  Value=0
  Relational Operator : RelationalOperator  Operator=>  RndMeth=Nearest  InputSameDT=on
  Out1 : Outport
  wires:
  Relational Operator/1 -> Out1/1
  In1/1 -> Relational Operator/1
  Constant4/1 -> Relational Operator/2

== system VCO_15N_2nd_order_2020a_v2/15-Stage Ring Oscillator1/Convert to Square Wave3 ==
  In1 : Inport
  Constant4 : Constant  Value=0
  Relational Operator : RelationalOperator  Operator=>  RndMeth=Nearest  InputSameDT=on
  Out1 : Outport
  wires:
  Relational Operator/1 -> Out1/1
  In1/1 -> Relational Operator/1
  Constant4/1 -> Relational Operator/2

== system VCO_15N_2nd_order_2020a_v2/15-Stage Ring Oscillator1/Convert to Square Wave4 ==
  In1 : Inport
  Constant4 : Constant  Value=0
  Relational Operator : RelationalOperator  Operator=>  RndMeth=Nearest  InputSameDT=on
  Out1 : Outport
  wires:
  Relational Operator/1 -> Out1/1
  In1/1 -> Relational Operator/1
  Constant4/1 -> Relational Operator/2

== system VCO_15N_2nd_order_2020a_v2/15-Stage Ring Oscillator1/Convert to Square Wave5 ==
  In1 : Inport
  Constant4 : Constant  Value=0
  Relational Operator : RelationalOperator  Operator=>  RndMeth=Nearest  InputSameDT=on
  Out1 : Outport
  wires:
  Relational Operator/1 -> Out1/1
  In1/1 -> Relational Operator/1
  Constant4/1 -> Relational Operator/2

== system VCO_15N_2nd_order_2020a_v2/15-Stage Ring Oscillator1/Convert to Square Wave6 ==
  In1 : Inport
  Constant4 : Constant  Value=0
  Relational Operator : RelationalOperator  Operator=>  RndMeth=Nearest  InputSameDT=on
  Out1 : Outport
  wires:
  Relational Operator/1 -> Out1/1
  In1/1 -> Relational Operator/1
  Constant4/1 -> Relational Operator/2

== system VCO_15N_2nd_order_2020a_v2/15-Stage Ring Oscillator1/Convert to Square Wave7 ==
  In1 : Inport
  Constant4 : Constant  Value=0
  Relational Operator : RelationalOperator  Operator=>  RndMeth=Nearest  InputSameDT=on
  Out1 : Outport
  wires:
  Relational Operator/1 -> Out1/1
  In1/1 -> Relational Operator/1
  Constant4/1 -> Relational Operator/2

== system VCO_15N_2nd_order_2020a_v2/15-Stage Ring Oscillator1/Convert to Square Wave8 ==
  In1 : Inport
  Constant4 : Constant  Value=0
  Relational Operator : RelationalOperator  Operator=>  RndMeth=Nearest  InputSameDT=on
  Out1 : Outport
  wires:
  Relational Operator/1 -> Out1/1
  In1/1 -> Relational Operator/1
  Constant4/1 -> Relational Operator/2

== system VCO_15N_2nd_order_2020a_v2/15-Stage Ring Oscillator1/Convert to Square Wave9 ==
  In1 : Inport
  Constant4 : Constant  Value=0
  Relational Operator : RelationalOperator  Operator=>  RndMeth=Nearest  InputSameDT=on
  Out1 : Outport
  wires:
  Relational Operator/1 -> Out1/1
  In1/1 -> Relational Operator/1
  Constant4/1 -> Relational Operator/2

== system VCO_15N_2nd_order_2020a_v2/15-Stage Ring Oscillator2/Convert to Square Wave ==
  In1 : Inport
  Constant4 : Constant  Value=0
  Relational Operator : RelationalOperator  Operator=>  RndMeth=Nearest  InputSameDT=on
  Out1 : Outport
  wires:
  Relational Operator/1 -> Out1/1
  In1/1 -> Relational Operator/1
  Constant4/1 -> Relational Operator/2

== system VCO_15N_2nd_order_2020a_v2/15-Stage Ring Oscillator2/Convert to Square Wave1 ==
  In1 : Inport
  Constant4 : Constant  Value=0
  Relational Operator : RelationalOperator  Operator=>  RndMeth=Nearest  InputSameDT=on
  Out1 : Outport
  wires:
  Relational Operator/1 -> Out1/1
  In1/1 -> Relational Operator/1
  Constant4/1 -> Relational Operator/2

== system VCO_15N_2nd_order_2020a_v2/15-Stage Ring Oscillator2/Convert to Square Wave10 ==
  In1 : Inport
  Constant4 : Constant  Value=0
  Relational Operator : RelationalOperator  Operator=>  RndMeth=Nearest  InputSameDT=on
  Out1 : Outport
  wires:
  Relational Operator/1 -> Out1/1
  In1/1 -> Relational Operator/1
  Constant4/1 -> Relational Operator/2

== system VCO_15N_2nd_order_2020a_v2/15-Stage Ring Oscillator2/Convert to Square Wave11 ==
  In1 : Inport
  Constant4 : Constant  Value=0
  Relational Operator : RelationalOperator  Operator=>  RndMeth=Nearest  InputSameDT=on
  Out1 : Outport
  wires:
  Relational Operator/1 -> Out1/1
  In1/1 -> Relational Operator/1
  Constant4/1 -> Relational Operator/2

== system VCO_15N_2nd_order_2020a_v2/15-Stage Ring Oscillator2/Convert to Square Wave12 ==
  In1 : Inport
  Constant4 : Constant  Value=0
  Relational Operator : RelationalOperator  Operator=>  RndMeth=Nearest  InputSameDT=on
  Out1 : Outport
  wires:
  Relational Operator/1 -> Out1/1
  In1/1 -> Relational Operator/1
  Constant4/1 -> Relational Operator/2

== system VCO_15N_2nd_order_2020a_v2/15-Stage Ring Oscillator2/Convert to Square Wave14 ==
  In1 : Inport
  Constant4 : Constant  Value=0
  Relational Operator : RelationalOperator  Operator=>  RndMeth=Nearest  InputSameDT=on
  Out1 : Outport
  wires:
  Relational Operator/1 -> Out1/1
  In1/1 -> Relational Operator/1
  Constant4/1 -> Relational Operator/2

== system VCO_15N_2nd_order_2020a_v2/15-Stage Ring Oscillator2/Convert to Square Wave15 ==
  In1 : Inport
  Constant4 : Constant  Value=0
  Relational Operator : RelationalOperator  Operator=>  RndMeth=Nearest  InputSameDT=on
  Out1 : Outport
  wires:
  Relational Operator/1 -> Out1/1
  In1/1 -> Relational Operator/1
  Constant4/1 -> Relational Operator/2

== system VCO_15N_2nd_order_2020a_v2/15-Stage Ring Oscillator2/Convert to Square Wave2 ==
  In1 : Inport
  Constant4 : Constant  Value=0
  Relational Operator : RelationalOperator  Operator=>  RndMeth=Nearest  InputSameDT=on
  Out1 : Outport
  wires:
  Relational Operator/1 -> Out1/1
  In1/1 -> Relational Operator/1
  Constant4/1 -> Relational Operator/2

== system VCO_15N_2nd_order_2020a_v2/15-Stage Ring Oscillator2/Convert to Square Wave3 ==
  In1 : Inport
  Constant4 : Constant  Value=0
  Relational Operator : RelationalOperator  Operator=>  RndMeth=Nearest  InputSameDT=on
  Out1 : Outport
  wires:
  Relational Operator/1 -> Out1/1
  In1/1 -> Relational Operator/1
  Constant4/1 -> Relational Operator/2

== system VCO_15N_2nd_order_2020a_v2/15-Stage Ring Oscillator2/Convert to Square Wave4 ==
  In1 : Inport
  Constant4 : Constant  Value=0
  Relational Operator : RelationalOperator  Operator=>  RndMeth=Nearest  InputSameDT=on
  Out1 : Outport
  wires:
  Relational Operator/1 -> Out1/1
  In1/1 -> Relational Operator/1
  Constant4/1 -> Relational Operator/2

== system VCO_15N_2nd_order_2020a_v2/15-Stage Ring Oscillator2/Convert to Square Wave5 ==
  In1 : Inport
  Constant4 : Constant  Value=0
  Relational Operator : RelationalOperator  Operator=>  RndMeth=Nearest  InputSameDT=on
  Out1 : Outport
  wires:
  Relational Operator/1 -> Out1/1
  In1/1 -> Relational Operator/1
  Constant4/1 -> Relational Operator/2

== system VCO_15N_2nd_order_2020a_v2/15-Stage Ring Oscillator2/Convert to Square Wave6 ==
  In1 : Inport
  Constant4 : Constant  Value=0
  Relational Operator : RelationalOperator  Operator=>  RndMeth=Nearest  InputSameDT=on
  Out1 : Outport
  wires:
  Relational Operator/1 -> Out1/1
  In1/1 -> Relational Operator/1
  Constant4/1 -> Relational Operator/2

== system VCO_15N_2nd_order_2020a_v2/15-Stage Ring Oscillator2/Convert to Square Wave7 ==
  In1 : Inport
  Constant4 : Constant  Value=0
  Relational Operator : RelationalOperator  Operator=>  RndMeth=Nearest  InputSameDT=on
  Out1 : Outport
  wires:
  Relational Operator/1 -> Out1/1
  In1/1 -> Relational Operator/1
  Constant4/1 -> Relational Operator/2

== system VCO_15N_2nd_order_2020a_v2/15-Stage Ring Oscillator2/Convert to Square Wave8 ==
  In1 : Inport
  Constant4 : Constant  Value=0
  Relational Operator : RelationalOperator  Operator=>  RndMeth=Nearest  InputSameDT=on
  Out1 : Outport
  wires:
  Relational Operator/1 -> Out1/1
  In1/1 -> Relational Operator/1
  Constant4/1 -> Relational Operator/2

== system VCO_15N_2nd_order_2020a_v2/15-Stage Ring Oscillator2/Convert to Square Wave9 ==
  In1 : Inport
  Constant4 : Constant  Value=0
  Relational Operator : RelationalOperator  Operator=>  RndMeth=Nearest  InputSameDT=on
  Out1 : Outport
  wires:
  Relational Operator/1 -> Out1/1
  In1/1 -> Relational Operator/1
  Constant4/1 -> Relational Operator/2

== system VCO_15N_2nd_order_2020a_v2/15-Stage Ring Oscillator3/Convert to Square Wave ==
  In1 : Inport
  Constant4 : Constant  Value=0
  Relational Operator : RelationalOperator  Operator=>  RndMeth=Nearest  InputSameDT=on
  Out1 : Outport
  wires:
  Relational Operator/1 -> Out1/1
  In1/1 -> Relational Operator/1
  Constant4/1 -> Relational Operator/2

== system VCO_15N_2nd_order_2020a_v2/15-Stage Ring Oscillator3/Convert to Square Wave1 ==
  In1 : Inport
  Constant4 : Constant  Value=0
  Relational Operator : RelationalOperator  Operator=>  RndMeth=Nearest  InputSameDT=on
  Out1 : Outport
  wires:
  Relational Operator/1 -> Out1/1
  In1/1 -> Relational Operator/1
  Constant4/1 -> Relational Operator/2

== system VCO_15N_2nd_order_2020a_v2/15-Stage Ring Oscillator3/Convert to Square Wave10 ==
  In1 : Inport
  Constant4 : Constant  Value=0
  Relational Operator : RelationalOperator  Operator=>  RndMeth=Nearest  InputSameDT=on
  Out1 : Outport
  wires:
  Relational Operator/1 -> Out1/1
  In1/1 -> Relational Operator/1
  Constant4/1 -> Relational Operator/2

== system VCO_15N_2nd_order_2020a_v2/15-Stage Ring Oscillator3/Convert to Square Wave11 ==
  In1 : Inport
  Constant4 : Constant  Value=0
  Relational Operator : RelationalOperator  Operator=>  RndMeth=Nearest  InputSameDT=on
  Out1 : Outport
  wires:
  Relational Operator/1 -> Out1/1
  In1/1 -> Relational Operator/1
  Constant4/1 -> Relational Operator/2

== system VCO_15N_2nd_order_2020a_v2/15-Stage Ring Oscillator3/Convert to Square Wave12 ==
  In1 : Inport
  Constant4 : Constant  Value=0
  Relational Operator : RelationalOperator  Operator=>  RndMeth=Nearest  InputSameDT=on
  Out1 : Outport
  wires:
  Relational Operator/1 -> Out1/1
  In1/1 -> Relational Operator/1
  Constant4/1 -> Relational Operator/2

== system VCO_15N_2nd_order_2020a_v2/15-Stage Ring Oscillator3/Convert to Square Wave14 ==
  In1 : Inport
  Constant4 : Constant  Value=0
  Relational Operator : RelationalOperator  Operator=>  RndMeth=Nearest  InputSameDT=on
  Out1 : Outport
  wires:
  Relational Operator/1 -> Out1/1
  In1/1 -> Relational Operator/1
  Constant4/1 -> Relational Operator/2

== system VCO_15N_2nd_order_2020a_v2/15-Stage Ring Oscillator3/Convert to Square Wave15 ==
  In1 : Inport
  Constant4 : Constant  Value=0
  Relational Operator : RelationalOperator  Operator=>  RndMeth=Nearest  InputSameDT=on
  Out1 : Outport
  wires:
  Relational Operator/1 -> Out1/1
  In1/1 -> Relational Operator/1
  Constant4/1 -> Relational Operator/2

== system VCO_15N_2nd_order_2020a_v2/15-Stage Ring Oscillator3/Convert to Square Wave2 ==
  In1 : Inport
  Constant4 : Constant  Value=0
  Relational Operator : RelationalOperator  Operator=>  RndMeth=Nearest  InputSameDT=on
  Out1 : Outport
  wires:
  Relational Operator/1 -> Out1/1
  In1/1 -> Relational Operator/1
  Constant4/1 -> Relational Operator/2

== system VCO_15N_2nd_order_2020a_v2/15-Stage Ring Oscillator3/Convert to Square Wave3 ==
  In1 : Inport
  Constant4 : Constant  Value=0
  Relational Operator : RelationalOperator  Operator=>  RndMeth=Nearest  InputSameDT=on
  Out1 : Outport
  wires:
  Relational Operator/1 -> Out1/1
  In1/1 -> Relational Operator/1
  Constant4/1 -> Relational Operator/2

== system VCO_15N_2nd_order_2020a_v2/15-Stage Ring Oscillator3/Convert to Square Wave4 ==
  In1 : Inport
  Constant4 : Constant  Value=0
  Relational Operator : RelationalOperator  Operator=>  RndMeth=Nearest  InputSameDT=on
  Out1 : Outport
  wires:
  Relational Operator/1 -> Out1/1
  In1/1 -> Relational Operator/1
  Constant4/1 -> Relational Operator/2

== system VCO_15N_2nd_order_2020a_v2/15-Stage Ring Oscillator3/Convert to Square Wave5 ==
  In1 : Inport
  Constant4 : Constant  Value=0
  Relational Operator : RelationalOperator  Operator=>  RndMeth=Nearest  InputSameDT=on
  Out1 : Outport
  wires:
  Relational Operator/1 -> Out1/1
  In1/1 -> Relational Operator/1
  Constant4/1 -> Relational Operator/2

== system VCO_15N_2nd_order_2020a_v2/15-Stage Ring Oscillator3/Convert to Square Wave6 ==
  In1 : Inport
  Constant4 : Constant  Value=0
  Relational Operator : RelationalOperator  Operator=>  RndMeth=Nearest  InputSameDT=on
  Out1 : Outport
  wires:
  Relational Operator/1 -> Out1/1
  In1/1 -> Relational Operator/1
  Constant4/1 -> Relational Operator/2

== system VCO_15N_2nd_order_2020a_v2/15-Stage Ring Oscillator3/Convert to Square Wave7 ==
  In1 : Inport
  Constant4 : Constant  Value=0
  Relational Operator : RelationalOperator  Operator=>  RndMeth=Nearest  InputSameDT=on
  Out1 : Outport
  wires:
  Relational Operator/1 -> Out1/1
  In1/1 -> Relational Operator/1
  Constant4/1 -> Relational Operator/2

== system VCO_15N_2nd_order_2020a_v2/15-Stage Ring Oscillator3/Convert to Square Wave8 ==
  In1 : Inport
  Constant4 : Constant  Value=0
  Relational Operator : RelationalOperator  Operator=>  RndMeth=Nearest  InputSameDT=on
  Out1 : Outport
  wires:
  Relational Operator/1 -> Out1/1
  In1/1 -> Relational Operator/1
  Constant4/1 -> Relational Operator/2

== system VCO_15N_2nd_order_2020a_v2/15-Stage Ring Oscillator3/Convert to Square Wave9 ==
  In1 : Inport
  Constant4 : Constant  Value=0
  Relational Operator : RelationalOperator  Operator=>  RndMeth=Nearest  InputSameDT=on
  Out1 : Outport
  wires:
  Relational Operator/1 -> Out1/1
  In1/1 -> Relational Operator/1
  Constant4/1 -> Relational Operator/2

== system VCO_15N_2nd_order_2020a_v2/15-Stage Ring Oscillator4/Convert to Square Wave ==
  In1 : Inport
  Constant4 : Constant  Value=0
  Relational Operator : RelationalOperator  Operator=>  RndMeth=Nearest  InputSameDT=on
  Out1 : Outport
  wires:
  Relational Operator/1 -> Out1/1
  In1/1 -> Relational Operator/1
  Constant4/1 -> Relational Operator/2
